simulink model "downsampletest"  (Simulink 6.2)
settings: Solver=ode45  StartTime=0.0  StopTime=50  RelTol=1e-3
libraries: xbsIndex_r3 x43, simulink x2
settings Model: LastModifiedBy=mdexter
settings DebuggingCC: SolverPrmCheckMsg=warning

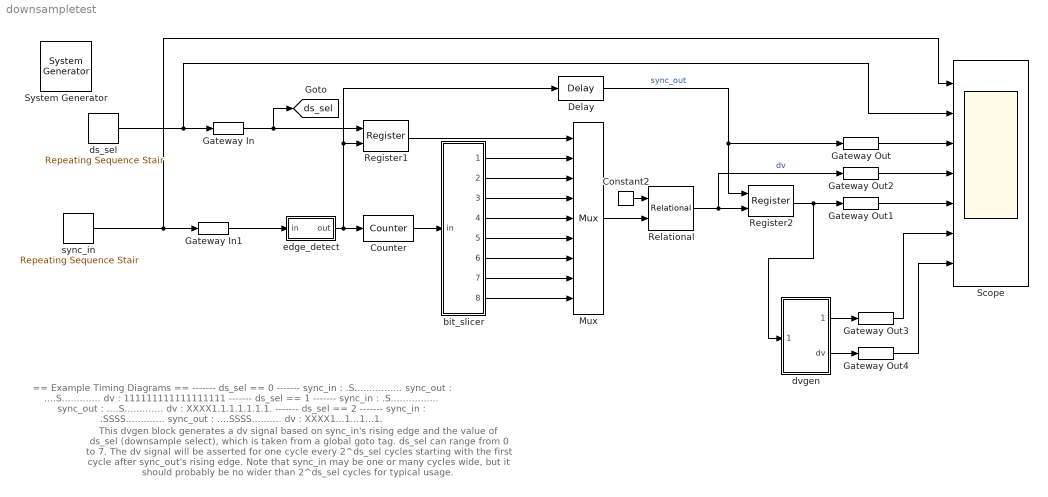
== system downsampletest ==
  note: This dvgen block generates a dv signal based on sync_in's rising
      | edge and the value of ds_sel (downsample select), which is taken
      | from a global goto tag.  ds_sel can range from 0 to 7.  The dv
      | signal will be asserted for one cycle every 2^ds_sel cycles starting
      | with the first cycle after sync_out's rising edge.  Note that sync_in
      | may be one or many cycles wide, but it should probably be no
      | wider than 2^ds_sel cycles for typical usage.
  note: == Example Timing Diagrams ==
      |
      | -------  ds_sel == 0  -------
      | sync_in : .S................
      | sync_out : ....S.............
      | dv : 111111111111111111
      |
      | -------  ds_sel == 1  -------
      | sync_in : .S................
      | sync_out : ....S.............
      | dv : XXXX1.1.1.1.1.1.1.
      |
      | -------  ds_sel == 2  -------
      | sync_in : .SSSS.............
      | sync_out : ....SSSS..........
      | dv : XXXX1...1...1...1.
  " System Generator" : xbsIndex_r3/ System Generator  Tag=genX  xilinxfamily=Virtex2P  part=xc2vp40  speed=-6  package=ff1152  synthesis_tool=XST  directory=./netlist  testbench=off  simulink_period=1  sysclk_period=100  incr_netlist=off  trim_vbits=Everywhere in SubSystem  dbl_ovrd=According to Block Masks  core_generation=According to Block Masks  run_coregen=off  deprecated_control=off  eval_field=0
      settings: AttributesFormatString=System\nGenerator
  Constant2 : xbsIndex_r3/Constant  const=0  equ=P=C  arith_type=Unsigned  n_bits=1  bin_pt=0  opselect=C  inp2=PCIN>>17  opr=+  inp1=P  carry=CIN  iostate=0  explicit_period=on  period=1  dbl_ovrd=off
  Counter : xbsIndex_r3/Counter  cnt_type=Free Running  n_bits=7  bin_pt=0  arith_type=Unsigned  start_count=0  cnt_to=Inf  cnt_by_val=1  operation=Up  explicit_period=off  period=1  load_pin=off  rst=on  en=off  dbl_ovrd=off  show_param=on  use_rpm=on  gen_core=off
      settings: xl_area=[0, 0, 0, 0, 0, 0, 0]
  Delay : xbsIndex_r3/Delay  latency=3  reg_retiming=off  explicit_period=off  period=1  en=off  accept_only_valid=off  init_zero=on  dbl_ovrd=off  show_param=off
      settings: xl_area=[0, 0, 0, 0, 0, 0, 0]
  Gateway In : xbsIndex_r3/Gateway In  arith_type=Unsigned  n_bits=3  bin_pt=0  quantization=Truncate  overflow=Wrap  period=1  timing_constraint=None  locs_specified=off  LOCs={}  needs_fixed_name=off  dbl_ovrd=off  show_param=off
      settings: xl_area=[0, 0, 0, 0, 0, 0, 0]
  Gateway In1 : xbsIndex_r3/Gateway In  arith_type=Boolean  n_bits=8  bin_pt=6  quantization=Truncate  overflow=Wrap  period=1  timing_constraint=None  locs_specified=off  LOCs={}  needs_fixed_name=off  dbl_ovrd=off  show_param=off
      settings: xl_area=[0, 0, 0, 0, 0, 0, 0]
  Gateway Out{,1..4} (5 alike) : xbsIndex_r3/Gateway Out  output_type=Double  nbits=8  bin_pt=6  arith_type=Boolean  quantization=Truncate  overflow=Wrap  hdl_port=on  timing_constraint=None  locs_specified=off  LOCs={}  needs_fixed_name=off  show_param=off
      settings: xl_area=[0, 0, 0, 0, 0, 0, 0]
  Mux : xbsIndex_r3/Mux  inputs=8  precision=Full  arith_type="Signed  (2's comp)"  n_bits=8  bin_pt=2  quantization=Truncate  overflow=Wrap  latency=1  explicit_period=off  period=1  en=off  dbl_ovrd=off  show_param=off  mux_type=off  use_rpm=off  gen_core=off
      settings: xl_area=[0, 0, 0, 0, 0, 0, 0]
  Register1 : xbsIndex_r3/Register  init=0  reg_only_valid=off  explicit_period=off  period=1  rst=off  en=on  out_en=off  dbl_ovrd=off  show_param=off
      settings: xl_area=[0, 0, 0, 0, 0, 0, 0]
  Register2 : xbsIndex_r3/Register  init=0  reg_only_valid=off  explicit_period=off  period=1  rst=off  en=on  out_en=off  dbl_ovrd=off  show_param=off
      settings: xl_area=[0, 0, 0, 0, 0, 0, 0]
  Relational : xbsIndex_r3/Relational  mode=a=b  latency=1  explicit_period=off  period=1  en=off  dbl_ovrd=off  show_param=on
      settings: xl_area=[0, 0, 0, 0, 0, 0, 0]
  Scope : Scope  NumInputPorts=7
      settings: YMin=-5~-5~-5~-5~-5~-5~-5  YMax=5~5~5~5~5~5~5
  bit_slicer : Subsystem
  ds_sel : simulink/Sources/Repeating Sequence Stair  OutValues=[0 0 zeros(1,8) 1*ones(1,19) zeros(1,1000)]  tsamp=-1  OutputDataTypeScalingMode=Specify via dialog  OutDataType=float('double')  ConRadixGroup=Best Precision: Vector-wise  OutScaling=2^-12
  dvgen : Subsystem
      settings: AttributesFormatString=Latency=3
  edge_detect : Subsystem  mask(Edge Detector){edge=Rising, polarity=Active High, xin=floor([0.5:0.5:5])*0.08, yin={[-1,-1,1,1,1,1,1,1,1,1],[1,1,-1,-1,-1,-1,-1,-1,-1,-1],[-1,-1,1,1,1,1,-1,-1,-1,-1]}, xout=1-floor([5:-0.5:0.5])*0.08, yout={[-1,-1,1,1,-1,-1,-1,-1,-1,-1],[-1,-1,1,1,-1,-1,-1,-1,-1,-1],[-1,-1,1,1,-1,-1,1,1,-1,-1]}}
      mask prompts: edge "Edge Type"; polarity "Output Polarity"; xin "Input X Positions"; yin "Input Y Positions"; xout "Output X Positions"; yout "Output Y Positions"
      mask help: Output is active for one-cycle after each edge of the specified type (i.e. rising, falling or both).
      mask init:
      | edge_detect_init(gcb,edge,polarity);
      settings: AttributesFormatString=|
      | rising edge
      | active high
      mask Help: Output is active for one-cycle after each edge of the specified type (i.e. rising, falling, or both).  Latency is zero.
      mask StyleString: popup(Rising|Falling|Both),popup(Active High|Active Low),edit,edit,edit,edit
      mask Display:
      | plot(xin,0.5+yin{edge}*0.2)
      | plot(xout,0.5+yout{edge}*0.2*(3-2*polarity))
  sync_in : simulink/Sources/Repeating Sequence Stair  OutValues=[0 1 zeros(1,6)]  tsamp=-1  OutputDataTypeScalingMode=Specify via dialog  OutDataType=float('double')  ConRadixGroup=Best Precision: Vector-wise  OutScaling=2^-12
  tag scope: ds_sel=global
  wires:
  bit_slicer/1(zero) -> Mux/2
  bit_slicer/2(b0_0) -> Mux/3
  bit_slicer/3(b1_0) -> Mux/4
  bit_slicer/4(b2_0) -> Mux/5
  bit_slicer/5(b3_0) -> Mux/6
  bit_slicer/6(b4_0) -> Mux/7
  bit_slicer/7(b5_0) -> Mux/8
  bit_slicer/8(b6_0) -> Mux/9
  Counter/1 -> bit_slicer/1(in)
  Mux/1 -> Relational/2
  Gateway In1/1 -> edge_detect/1(in)
  Constant2/1 -> Relational/1
  edge_detect/1(out) -> Counter/1, Register1/2, Delay/1
  Delay/1 -> Gateway Out/1, Register2/1  "sync_out"
  Relational/1 -> Gateway Out2/1, Register2/2  "dv"
  sync_in/1 -> Gateway In1/1, Scope/1
  Register2/1 -> Gateway Out1/1, dvgen/1(sync_in)
  Gateway Out/1 -> Scope/3
  ds_sel/1 -> Gateway In/1, Scope/2
  dvgen/1(sync_out) -> Gateway Out3/1
  dvgen/2(dv) -> Gateway Out4/1
  Gateway Out3/1 -> Scope/6
  Gateway Out4/1 -> Scope/7
  Register1/1 -> Mux/1
  Gateway In/1 -> Register1/1, [ds_sel]
  Gateway Out1/1 -> Scope/5
  Gateway Out2/1 -> Scope/4

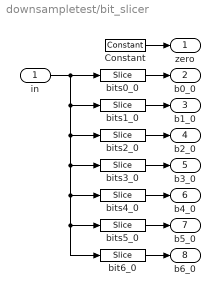
== system downsampletest/bit_slicer ==
  in : Inport  Port=1  LatchInput=off
  Constant : xbsIndex_r3/Constant  const=0  equ=P=C  arith_type=Unsigned  n_bits=1  bin_pt=0  opselect=C  inp2=PCIN>>17  opr=+  inp1=P  carry=CIN  iostate=0  explicit_period=on  period=1  dbl_ovrd=off
  bit6_0 : xbsIndex_r3/Slice  mode=Lower Bit Location + Width  nbits=7  bit1=0  base1=MSB of Input  bit0=0  base0=LSB of Input  boolean_output=off  explicit_period=off  period=1  dbl_ovrd=off
  bits0_0 : xbsIndex_r3/Slice  mode=Lower Bit Location + Width  nbits=1  bit1=0  base1=MSB of Input  bit0=0  base0=LSB of Input  boolean_output=off  explicit_period=off  period=1  dbl_ovrd=off
  bits1_0 : xbsIndex_r3/Slice  mode=Lower Bit Location + Width  nbits=2  bit1=0  base1=MSB of Input  bit0=0  base0=LSB of Input  boolean_output=off  explicit_period=off  period=1  dbl_ovrd=off
  bits2_0 : xbsIndex_r3/Slice  mode=Lower Bit Location + Width  nbits=3  bit1=0  base1=MSB of Input  bit0=0  base0=LSB of Input  boolean_output=off  explicit_period=off  period=1  dbl_ovrd=off
  bits3_0 : xbsIndex_r3/Slice  mode=Lower Bit Location + Width  nbits=4  bit1=0  base1=MSB of Input  bit0=0  base0=LSB of Input  boolean_output=off  explicit_period=off  period=1  dbl_ovrd=off
  bits4_0 : xbsIndex_r3/Slice  mode=Lower Bit Location + Width  nbits=5  bit1=0  base1=MSB of Input  bit0=0  base0=LSB of Input  boolean_output=off  explicit_period=off  period=1  dbl_ovrd=off
  bits5_0 : xbsIndex_r3/Slice  mode=Lower Bit Location + Width  nbits=6  bit1=0  base1=MSB of Input  bit0=0  base0=LSB of Input  boolean_output=off  explicit_period=off  period=1  dbl_ovrd=off
  zero : Outport
  b0_0 : Outport  Port=2
  b1_0 : Outport  Port=3
  b2_0 : Outport  Port=4
  b3_0 : Outport  Port=5
  b4_0 : Outport  Port=6
  b5_0 : Outport  Port=7
  b6_0 : Outport  Port=8
  wires:
  in/1 -> bits5_0/1, bit6_0/1, bits4_0/1, bits3_0/1, bits2_0/1, bits1_0/1, bits0_0/1
  bits0_0/1 -> b0_0/1
  bits1_0/1 -> b1_0/1
  bits2_0/1 -> b2_0/1
  bits3_0/1 -> b3_0/1
  bits4_0/1 -> b4_0/1
  bits5_0/1 -> b5_0/1
  bit6_0/1 -> b6_0/1
  Constant/1 -> zero/1

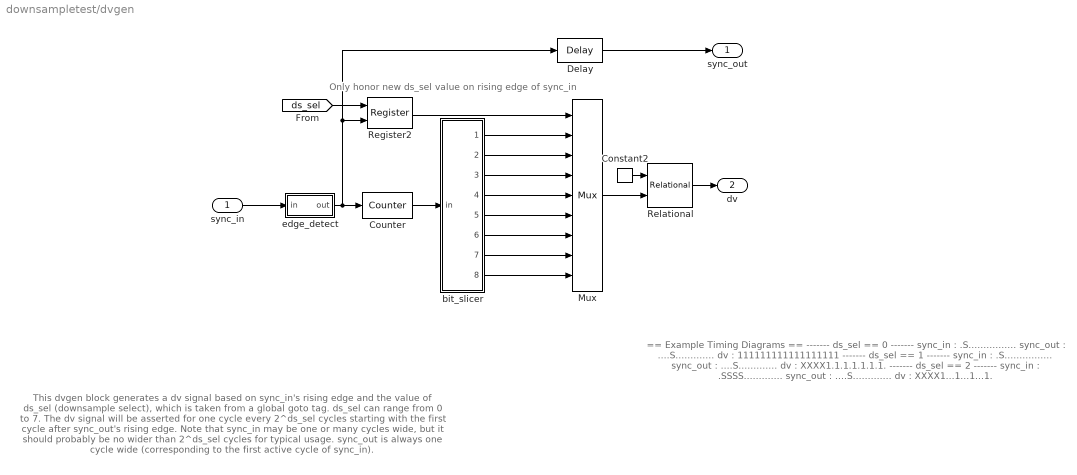
== system downsampletest/dvgen ==
  note: This dvgen block generates a dv signal based on sync_in's rising
      | edge and the value of ds_sel (downsample select), which is taken
      | from a global goto tag.  ds_sel can range from 0 to 7.  The dv
      | signal will be asserted for one cycle every 2^ds_sel cycles starting
      | with the first cycle after sync_out's rising edge.  Note that sync_in
      | may be one or many cycles wide, but it should probably be no
      | wider than 2^ds_sel cycles for typical usage.  sync_out is always
      | one cycle wide (corresponding to the first active cycle of sync_in).
  note: == Example Timing Diagrams ==
      |
      | -------  ds_sel == 0  -------
      | sync_in : .S................
      | sync_out : ....S.............
      | dv : 111111111111111111
      |
      | -------  ds_sel == 1  -------
      | sync_in : .S................
      | sync_out : ....S.............
      | dv : XXXX1.1.1.1.1.1.1.
      |
      | -------  ds_sel == 2  -------
      | sync_in : .SSSS.............
      | sync_out : ....S.............
      | dv : XXXX1...1...1...1.
  note: Only honor new ds_sel value
      | on rising edge of sync_in
  sync_in : Inport  Port=1  LatchInput=off
  Constant2 : xbsIndex_r3/Constant  const=0  equ=P=C  arith_type=Unsigned  n_bits=1  bin_pt=0  opselect=C  inp2=PCIN>>17  opr=+  inp1=P  carry=CIN  iostate=0  explicit_period=on  period=1  dbl_ovrd=off
  Counter : xbsIndex_r3/Counter  cnt_type=Free Running  n_bits=7  bin_pt=0  arith_type=Unsigned  start_count=0  cnt_to=Inf  cnt_by_val=1  operation=Up  explicit_period=off  period=1  load_pin=off  rst=on  en=off  dbl_ovrd=off  show_param=on  use_rpm=on  gen_core=off
      settings: xl_area=[0, 0, 0, 0, 0, 0, 0]
  Delay : xbsIndex_r3/Delay  latency=3  reg_retiming=off  explicit_period=off  period=1  en=off  accept_only_valid=off  init_zero=on  dbl_ovrd=off  show_param=off
      settings: xl_area=[0, 0, 0, 0, 0, 0, 0]
  Mux : xbsIndex_r3/Mux  inputs=8  precision=Full  arith_type="Signed  (2's comp)"  n_bits=8  bin_pt=2  quantization=Truncate  overflow=Wrap  latency=1  explicit_period=off  period=1  en=off  dbl_ovrd=off  show_param=off  mux_type=off  use_rpm=off  gen_core=off
      settings: xl_area=[0, 0, 0, 0, 0, 0, 0]
  Register2 : xbsIndex_r3/Register  init=0  reg_only_valid=off  explicit_period=off  period=1  rst=off  en=on  out_en=off  dbl_ovrd=off  show_param=off
      settings: xl_area=[0, 0, 0, 0, 0, 0, 0]
  Relational : xbsIndex_r3/Relational  mode=a=b  latency=1  explicit_period=off  period=1  en=off  dbl_ovrd=off  show_param=on
      settings: xl_area=[0, 0, 0, 0, 0, 0, 0]
  bit_slicer : Subsystem
  edge_detect : Subsystem  mask(Edge Detector){edge=Rising, polarity=Active High, xin=floor([0.5:0.5:5])*0.08, yin={[-1,-1,1,1,1,1,1,1,1,1],[1,1,-1,-1,-1,-1,-1,-1,-1,-1],[-1,-1,1,1,1,1,-1,-1,-1,-1]}, xout=1-floor([5:-0.5:0.5])*0.08, yout={[-1,-1,1,1,-1,-1,-1,-1,-1,-1],[-1,-1,1,1,-1,-1,-1,-1,-1,-1],[-1,-1,1,1,-1,-1,1,1,-1,-1]}}
      mask prompts: edge "Edge Type"; polarity "Output Polarity"; xin "Input X Positions"; yin "Input Y Positions"; xout "Output X Positions"; yout "Output Y Positions"
      mask help: Output is active for one-cycle after each edge of the specified type (i.e. rising, falling or both).
      mask init:
      | edge_detect_init(gcb,edge,polarity);
      settings: AttributesFormatString=|
      | rising edge
      | active high
      mask Help: Output is active for one-cycle after each edge of the specified type (i.e. rising, falling, or both).  Latency is zero.
      mask StyleString: popup(Rising|Falling|Both),popup(Active High|Active Low),edit,edit,edit,edit
      mask Display:
      | plot(xin,0.5+yin{edge}*0.2)
      | plot(xout,0.5+yout{edge}*0.2*(3-2*polarity))
  sync_out : Outport
  dv : Outport  Port=2
  wires:
  bit_slicer/1(zero) -> Mux/2
  bit_slicer/2(b0_0) -> Mux/3
  bit_slicer/3(b1_0) -> Mux/4
  bit_slicer/4(b2_0) -> Mux/5
  bit_slicer/5(b3_0) -> Mux/6
  bit_slicer/6(b4_0) -> Mux/7
  bit_slicer/7(b5_0) -> Mux/8
  bit_slicer/8(b6_0) -> Mux/9
  Counter/1 -> bit_slicer/1(in)
  Register2/1 -> Mux/1
  Mux/1 -> Relational/2
  sync_in/1 -> edge_detect/1(in)
  Constant2/1 -> Relational/1
  edge_detect/1(out) -> Counter/1, Register2/2, Delay/1
  Delay/1 -> sync_out/1
  Relational/1 -> dv/1
  [ds_sel] -> Register2/1

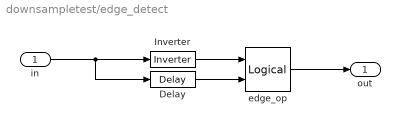
== system downsampletest/edge_detect ==
  in : Inport  Port=1  LatchInput=off
  Delay : xbsIndex_r3/Delay  latency=1  reg_retiming=off  explicit_period=off  period=1  en=off  accept_only_valid=off  init_zero=on  dbl_ovrd=off  show_param=off
      settings: xl_area=[0, 0, 0, 0, 0, 0, 0]
  Inverter : xbsIndex_r3/Inverter  latency=0  explicit_period=off  period=1  en=off  dbl_ovrd=off  show_param=off
      settings: xl_area=[0, 0, 0, 0, 0, 0, 0]
  edge_op : xbsIndex_r3/Logical  logical_function=NOR  inputs=2  precision=Full  arith_type=Unsigned  n_bits=8  bin_pt=2  align_bp=on  latency=0  explicit_period=off  period=1  en=off  dbl_ovrd=off  show_param=off
      settings: xl_area=[0, 0, 0, 0, 0, 0, 0]
  out : Outport
  wires:
  Delay/1 -> edge_op/2
  in/1 -> Delay/1, Inverter/1
  edge_op/1 -> out/1
  Inverter/1 -> edge_op/1

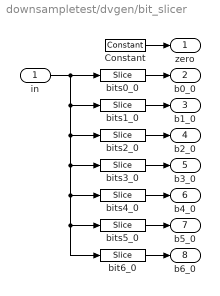
== system downsampletest/dvgen/bit_slicer ==
  in : Inport  Port=1  LatchInput=off
  Constant : xbsIndex_r3/Constant  const=0  equ=P=C  arith_type=Unsigned  n_bits=1  bin_pt=0  opselect=C  inp2=PCIN>>17  opr=+  inp1=P  carry=CIN  iostate=0  explicit_period=on  period=1  dbl_ovrd=off
  bit6_0 : xbsIndex_r3/Slice  mode=Lower Bit Location + Width  nbits=7  bit1=0  base1=MSB of Input  bit0=0  base0=LSB of Input  boolean_output=off  explicit_period=off  period=1  dbl_ovrd=off
  bits0_0 : xbsIndex_r3/Slice  mode=Lower Bit Location + Width  nbits=1  bit1=0  base1=MSB of Input  bit0=0  base0=LSB of Input  boolean_output=off  explicit_period=off  period=1  dbl_ovrd=off
  bits1_0 : xbsIndex_r3/Slice  mode=Lower Bit Location + Width  nbits=2  bit1=0  base1=MSB of Input  bit0=0  base0=LSB of Input  boolean_output=off  explicit_period=off  period=1  dbl_ovrd=off
  bits2_0 : xbsIndex_r3/Slice  mode=Lower Bit Location + Width  nbits=3  bit1=0  base1=MSB of Input  bit0=0  base0=LSB of Input  boolean_output=off  explicit_period=off  period=1  dbl_ovrd=off
  bits3_0 : xbsIndex_r3/Slice  mode=Lower Bit Location + Width  nbits=4  bit1=0  base1=MSB of Input  bit0=0  base0=LSB of Input  boolean_output=off  explicit_period=off  period=1  dbl_ovrd=off
  bits4_0 : xbsIndex_r3/Slice  mode=Lower Bit Location + Width  nbits=5  bit1=0  base1=MSB of Input  bit0=0  base0=LSB of Input  boolean_output=off  explicit_period=off  period=1  dbl_ovrd=off
  bits5_0 : xbsIndex_r3/Slice  mode=Lower Bit Location + Width  nbits=6  bit1=0  base1=MSB of Input  bit0=0  base0=LSB of Input  boolean_output=off  explicit_period=off  period=1  dbl_ovrd=off
  zero : Outport
  b0_0 : Outport  Port=2
  b1_0 : Outport  Port=3
  b2_0 : Outport  Port=4
  b3_0 : Outport  Port=5
  b4_0 : Outport  Port=6
  b5_0 : Outport  Port=7
  b6_0 : Outport  Port=8
  wires:
  in/1 -> bits5_0/1, bit6_0/1, bits4_0/1, bits3_0/1, bits2_0/1, bits1_0/1, bits0_0/1
  bits0_0/1 -> b0_0/1
  bits1_0/1 -> b1_0/1
  bits2_0/1 -> b2_0/1
  bits3_0/1 -> b3_0/1
  bits4_0/1 -> b4_0/1
  bits5_0/1 -> b5_0/1
  bit6_0/1 -> b6_0/1
  Constant/1 -> zero/1

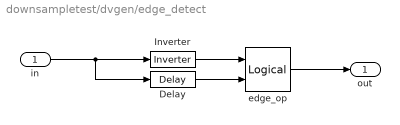
== system downsampletest/dvgen/edge_detect ==
  in : Inport  Port=1  LatchInput=off
  Delay : xbsIndex_r3/Delay  latency=1  reg_retiming=off  explicit_period=off  period=1  en=off  accept_only_valid=off  init_zero=on  dbl_ovrd=off  show_param=off
      settings: xl_area=[0, 0, 0, 0, 0, 0, 0]
  Inverter : xbsIndex_r3/Inverter  latency=0  explicit_period=off  period=1  en=off  dbl_ovrd=off  show_param=off
      settings: xl_area=[0, 0, 0, 0, 0, 0, 0]
  edge_op : xbsIndex_r3/Logical  logical_function=NOR  inputs=2  precision=Full  arith_type=Unsigned  n_bits=8  bin_pt=2  align_bp=on  latency=0  explicit_period=off  period=1  en=off  dbl_ovrd=off  show_param=off
      settings: xl_area=[0, 0, 0, 0, 0, 0, 0]
  out : Outport
  wires:
  Delay/1 -> edge_op/2
  in/1 -> Delay/1, Inverter/1
  edge_op/1 -> out/1
  Inverter/1 -> edge_op/1
